simulink library "AtmosphericModel"  (R2021b)
settings: Solver=VariableStepAuto  StartTime=0.0  StopTime=10.0  RelTol=1e-3
settings Model: Creator=setup  LastModifiedBy=dmgp1

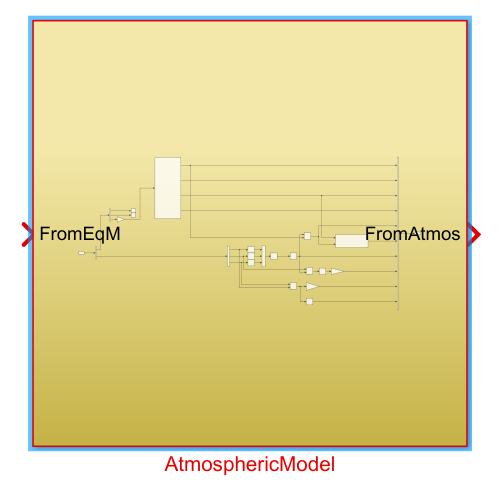
[thumbnail: Simulink's stored preview of the top-level diagram]
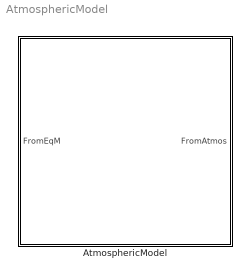
== system AtmosphericModel ==
  AtmosphericModel : Subsystem

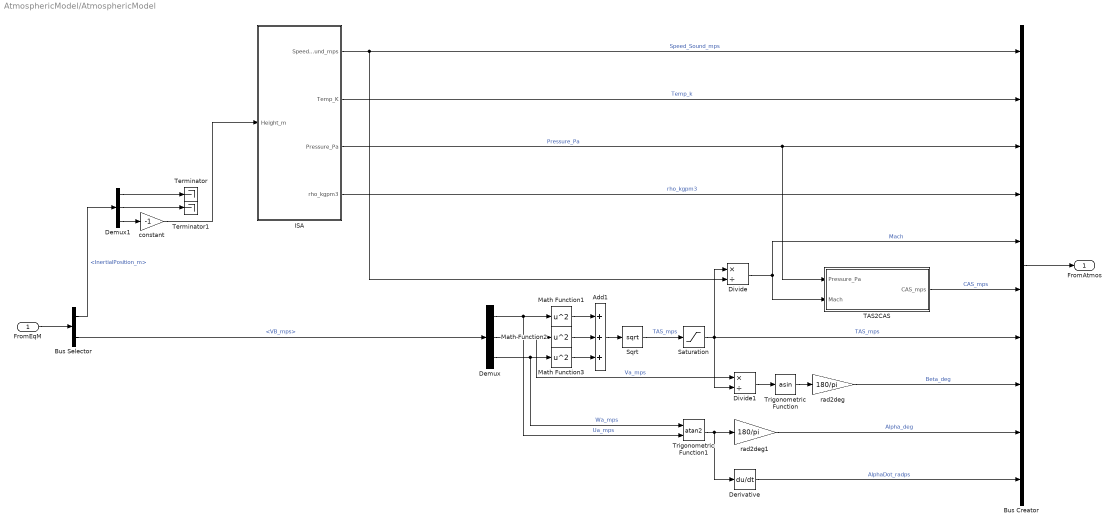
== system AtmosphericModel/AtmosphericModel ==
  FromEqM : Inport
  Add1 : Sum  Inputs=+++
  Bus Creator : BusCreator  Inputs=10
  Bus Selector : BusSelector  OutputSignals=InertialPosition_m,VB_mps
  Demux : Demux  Outputs=3
  Demux1 : Demux  Outputs=3
  Derivative : Derivative
  Divide : Product  Inputs=*/
  Divide1 : Product  Inputs=*/
  ISA : Subsystem
  Math Function1 : Math  Operator=square  SignedPower=on  SaturateOnIntegerOverflow=on
  Math Function2 : Math  Operator=square  SignedPower=on  SaturateOnIntegerOverflow=on
  Math Function3 : Math  Operator=square  SignedPower=on  SaturateOnIntegerOverflow=on
  Saturation : Saturate  UpperLimit=Inf  LowerLimit=0.1
  Sqrt : Sqrt  SaturateOnIntegerOverflow=on
  TAS2CAS : Subsystem
  Terminator : Terminator
  Terminator1 : Terminator
  Trigonometric Function : Trigonometry  Operator=asin
  Trigonometric Function1 : Trigonometry  Operator=atan2
  constant : Gain  Gain=-1
  rad2deg : Gain  Gain=180/pi
  rad2deg1 : Gain  Gain=180/pi
  FromAtmos : Outport
  wires:
  Saturation/1 -> Divide1/2, Bus Creator/7, Divide/1  "TAS_mps"
  ISA/3(Pressure_Pa) -> TAS2CAS/1(Pressure_Pa), Bus Creator/3  "Pressure_Pa"
  TAS2CAS/1(CAS_mps) -> Bus Creator/6  "CAS_mps"
  ISA/1(Speed_Sound_mps) -> Divide/2, Bus Creator/1  "Speed_Sound_mps"
  Trigonometric Function1/1 -> rad2deg1/1, Derivative/1
  Demux/2 -> Math Function2/1, Divide1/1  "Va_mps"
  ISA/2(Temp_K) -> Bus Creator/2  "Temp_k"
  Bus Selector/2 -> Demux/1  "<VB_mps>"
  Math Function2/1 -> Add1/2
  FromEqM/1 -> Bus Selector/1
  Math Function1/1 -> Add1/1
  Divide/1 -> Bus Creator/5, TAS2CAS/2(Mach)  "Mach"
  ISA/4(rho_kgpm3) -> Bus Creator/4  "rho_kgpm3"
  Derivative/1 -> Bus Creator/10  "AlphaDot_radps"
  rad2deg/1 -> Bus Creator/8  "Beta_deg"
  Math Function3/1 -> Add1/3
  Sqrt/1 -> Saturation/1  "TAS_mps"
  Demux/1 -> Math Function1/1, Trigonometric Function1/2  "Ua_mps"
  Trigonometric Function/1 -> rad2deg/1
  Demux/3 -> Math Function3/1, Trigonometric Function1/1  "Wa_mps"
  constant/1 -> ISA/1("Height_m ")
  rad2deg1/1 -> Bus Creator/9  "Alpha_deg"
  Divide1/1 -> Trigonometric Function/1
  Demux1/3 -> constant/1
  Demux1/1 -> Terminator/1
  Demux1/2 -> Terminator1/1
  Bus Creator/1 -> FromAtmos/1
  Bus Selector/1 -> Demux1/1  "<InertialPosition_m>"
  Add1/1 -> Sqrt/1

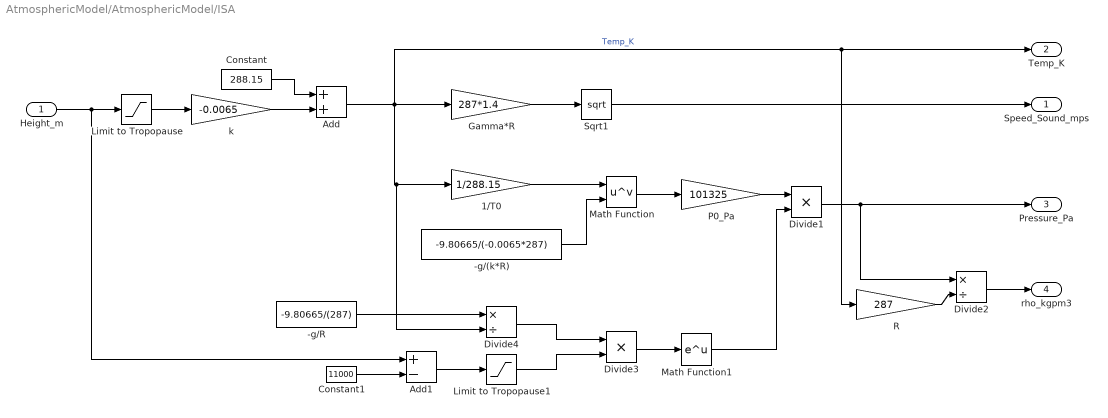
== system AtmosphericModel/AtmosphericModel/ISA ==
  "Height_m " : Inport
  -g/(k*R) : Constant  Value=-9.80665/(-0.0065*287)
  -g/R : Constant  Value=-9.80665/(287)
  1/T0 : Gain  Gain=1/288.15
  Add : Sum
  Add1 : Sum  Inputs=+-
  Constant : Constant  Value=288.15
  Constant1 : Constant  Value=11000
  Divide1 : Product  Inputs=**
  Divide2 : Product  Inputs=*/
  Divide3 : Product  Inputs=**
  Divide4 : Product  Inputs=*/
  Gamma*R : Gain  Gain=287*1.4
  Limit to Tropopause : Saturate  UpperLimit=11000  LowerLimit=0
  Limit to Tropopause1 : Saturate  UpperLimit=inf  LowerLimit=0
  Math Function : Math  Operator=pow  SignedPower=on  SaturateOnIntegerOverflow=on
  Math Function1 : Math  SignedPower=on  SaturateOnIntegerOverflow=on
  P0_Pa : Gain  Gain=101325
  R : Gain  Gain=287
  Sqrt1 : Sqrt  SaturateOnIntegerOverflow=on
  k : Gain  Gain=-0.0065
  Speed_Sound_mps : Outport
  Temp_K : Outport  Port=2
  Pressure_Pa : Outport  Port=3
  rho_kgpm3 : Outport  Port=4
  wires:
  Divide1/1 -> Pressure_Pa/1, Divide2/1
  Gamma*R/1 -> Sqrt1/1
  k/1 -> Add/2
  Add/1 -> Gamma*R/1, Temp_K/1, R/1, 1/T0/1, Divide4/2  "Temp_K"
  Add1/1 -> Limit to Tropopause1/1
  Limit to Tropopause/1 -> k/1
  Constant1/1 -> Add1/2
  Divide4/1 -> Divide3/1
  Constant/1 -> Add/1
  Math Function/1 -> P0_Pa/1
  P0_Pa/1 -> Divide1/1
  Limit to Tropopause1/1 -> Divide3/2
  R/1 -> Divide2/2
  Divide2/1 -> rho_kgpm3/1
  1/T0/1 -> Math Function/1
  -g/(k*R)/1 -> Math Function/2
  Math Function1/1 -> Divide1/2
  "Height_m "/1 -> Limit to Tropopause/1, Add1/1
  Sqrt1/1 -> Speed_Sound_mps/1
  -g/R/1 -> Divide4/1
  Divide3/1 -> Math Function1/1

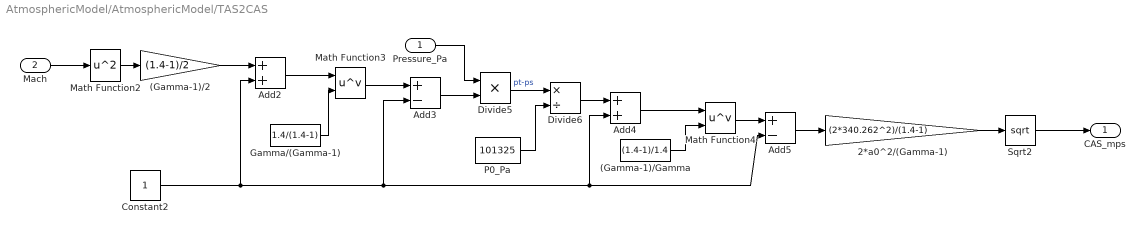
== system AtmosphericModel/AtmosphericModel/TAS2CAS ==
  Pressure_Pa : Inport
  Mach : Inport  Port=2
  (Gamma-1)/2 : Gain  Gain=(1.4-1)/2
  (Gamma-1)/Gamma : Constant  Value=(1.4-1)/1.4
  2*a0^2/(Gamma-1) : Gain  Gain=(2*340.262^2)/(1.4-1)
  Add2 : Sum
  Add3 : Sum  Inputs=+-
  Add4 : Sum
  Add5 : Sum  Inputs=+-
  Constant2 : Constant
  Divide5 : Product  Inputs=**
  Divide6 : Product  Inputs=*/
  Gamma/(Gamma-1) : Constant  Value=1.4/(1.4-1)
  Math Function2 : Math  Operator=square  SignedPower=on  SaturateOnIntegerOverflow=on
  Math Function3 : Math  Operator=pow  SignedPower=on  SaturateOnIntegerOverflow=on
  Math Function4 : Math  Operator=pow  SignedPower=on  SaturateOnIntegerOverflow=on
  P0_Pa : Constant  Value=101325
  Sqrt2 : Sqrt  SaturateOnIntegerOverflow=on
  CAS_mps : Outport
  wires:
  Divide6/1 -> Add4/1
  Constant2/1 -> Add2/2, Add3/2, Add4/2, Add5/2
  Math Function2/1 -> (Gamma-1)/2/1
  Sqrt2/1 -> CAS_mps/1
  Mach/1 -> Math Function2/1
  Gamma/(Gamma-1)/1 -> Math Function3/2
  2*a0^2/(Gamma-1)/1 -> Sqrt2/1
  Math Function3/1 -> Add3/1
  (Gamma-1)/2/1 -> Add2/1
  Add5/1 -> 2*a0^2/(Gamma-1)/1
  Math Function4/1 -> Add5/1
  Pressure_Pa/1 -> Divide5/1
  (Gamma-1)/Gamma/1 -> Math Function4/2
  Add2/1 -> Math Function3/1
  Add3/1 -> Divide5/2
  P0_Pa/1 -> Divide6/2
  Add4/1 -> Math Function4/1
  Divide5/1 -> Divide6/1  "pt-ps"
